simulink model "lunwen_huitu"  (R2020b)
settings: Solver=ode45  StartTime=0.0  StopTime=2  RelTol=1e-3  EnableMultiTasking=on
values from neighbouring files (symbols this model uses):
  alphar = poly2sym(y3,t)    [lpv_model.m]
  hr = poly2sym(y6,t)    [lpv_model.m]
  miur = poly2sym(y2,t)    [lpv_model.m]
  qr = poly2sym(y4,t)    [lpv_model.m]
  Vr = poly2sym(y1,t)    [lpv_model.m]
  xr = poly2sym(y5,t)    [lpv_model.m]    (also in xr(0.0.01.2).mat = [9.97354758391 9.97900733809 9.98348279699 9.98718538751 9.9)
settings Model: Creator=YuXiaozhi  LastModifiedBy=Eric
settings DataIOCC: LimitDataPoints=on  SaveFormat=Array  ReturnWorkspaceOutputs=off
settings OptimizationCC: LifeSpan=inf
settings DebuggingCC: SolverPrmCheckMsg=warning  SFUnexpectedBacktrackingDiag=warning  SFNoUnconditionalDefaultTransitionDiag=warning  ArithmeticOperatorsInVariantConditions=warning
settings HardwareCC: ProdBitPerPointer=32  ProdBitPerSizeT=32  ProdBitPerPtrDiffT=32  ProdLargestAtomicFloat=None  ProdIntDivRoundTo=Undefined  ProdEndianess=Unspecified  ProdWordSize=32  ProdHWDeviceType=32-bit Generic
settings ModelReferenceCC: PropagateSignalLabelsOutOfModel=off
settings SFSimCC: SimUseLocalCustomCode=off  CustomCodeUndefinedFunction=UseInterfaceOnly
settings RTWCC: RTWUseLocalCustomCode=off
settings CodeAppCC: StateflowObjectComments=on
settings GRTTargetCC: TargetLangStandard=C89/C90 (ANSI)
settings ConfigComp: CovMetricSettings=dw  CovSaveCumulativeToWorkspaceVar=on  CovSaveSingleToWorkspaceVar=on  CovExternalEMLEnable=off  CovSFcnEnable=off

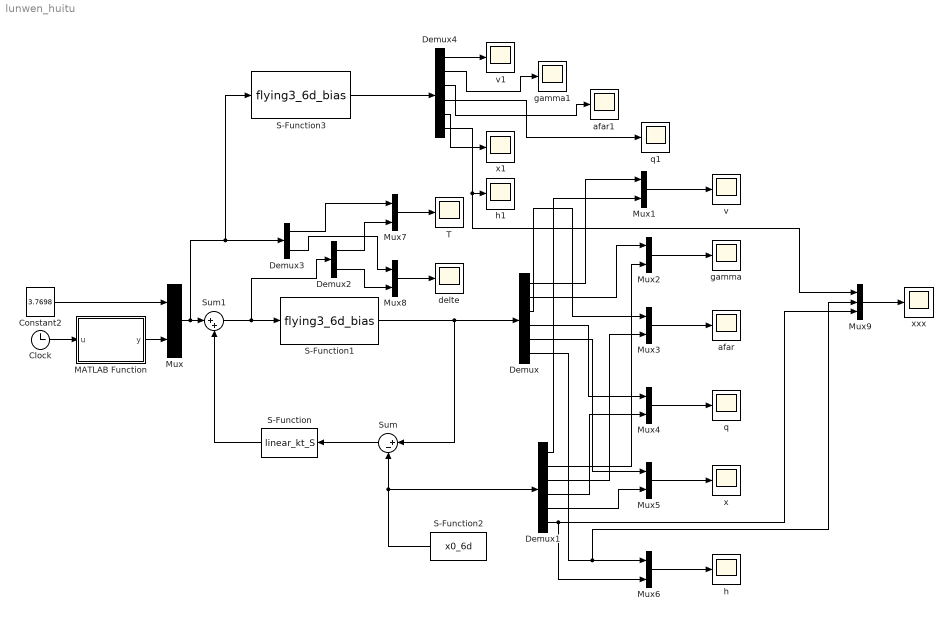
== system lunwen_huitu ==
  Clock : Clock
  Constant2 : Constant  Value=3.7698
  Demux : Demux  Outputs=6
  Demux1 : Demux  Outputs=6
  Demux2 : Demux  Outputs=2
  Demux3 : Demux  Outputs=2
  Demux4 : Demux  Outputs=6
  MATLAB Function : MATLAB Function  TreatAsAtomicUnit=on
  Mux{,1..8} (9 alike) : Mux  Inputs=2
  Mux9 : Mux  Inputs=3
  S-Function : S-Function  FunctionName=linear_kt_S  Parameters=Kall  SFunctionDeploymentMode=off  EnableBusSupport=off
  S-Function1 : S-Function  FunctionName=flying3_6d_bias  SFunctionDeploymentMode=off  EnableBusSupport=off
  S-Function2 : S-Function  FunctionName=x0_6d  Parameters=Vr,miur,alphar,qr,xr,hr  SFunctionDeploymentMode=off  EnableBusSupport=off
  S-Function3 : S-Function  FunctionName=flying3_6d_bias  SFunctionDeploymentMode=off  EnableBusSupport=off
  Sum : Sum  Inputs=|+-
  Sum1 : Sum  Inputs=|++
  T : Scope
  afar : Scope
  afar1 : Scope
  delte : Scope
  gamma : Scope
  gamma1 : Scope
  h : Scope
  h1 : Scope
  q : Scope
  q1 : Scope
  v : Scope
  v1 : Scope
  x : Scope
  x1 : Scope
  xxx : Scope
  wires:
  S-Function1/1 -> Sum/1, Demux/1
  S-Function2/1 -> Demux1/1, Sum/2
  Sum/1 -> S-Function/1
  Clock/1 -> MATLAB Function/1(u)
  Constant2/1 -> Mux/1
  MATLAB Function/1(y) -> Mux/2
  Mux/1 -> S-Function3/1, Demux3/1, Sum1/1
  Sum1/1 -> Demux2/1, S-Function1/1
  Demux2/1 -> Mux7/2
  Demux2/2 -> Mux8/2
  Mux7/1 -> T/1
  Mux8/1 -> delte/1
  Demux3/1 -> Mux7/1
  Demux3/2 -> Mux8/1
  Demux/1 -> Mux1/1
  Demux/2 -> Mux2/1
  Demux/3 -> Mux3/1
  Demux/4 -> Mux4/1
  Demux/5 -> Mux5/1
  Demux/6 -> Mux9/2, Mux6/1
  Demux1/1 -> Mux1/2
  Demux1/2 -> Mux2/2
  Demux1/3 -> Mux3/2
  Demux1/4 -> Mux4/2
  Demux1/5 -> Mux5/2
  Demux1/6 -> Mux9/3, Mux6/2
  Mux1/1 -> v/1
  Mux2/1 -> gamma/1
  Mux3/1 -> afar/1
  Mux4/1 -> q/1
  Mux5/1 -> x/1
  Mux6/1 -> h/1
  S-Function3/1 -> Demux4/1
  Demux4/1 -> v1/1
  Demux4/2 -> gamma1/1
  Demux4/3 -> afar1/1
  Demux4/4 -> q1/1
  Demux4/5 -> x1/1
  Demux4/6 -> Mux9/1, h1/1
  Mux9/1 -> xxx/1
  S-Function/1 -> Sum1/2

== matlab function lunwen_huitu/MATLAB Function ==
  data: u input; y output
function y = fcn(u)
if u<0.3
    y=-(11+(u)/0.3*22)/180*pi;
else if u>=0.3&&u<0.5
        y=-(33+(u-0.3)/0.2*15)/180*pi;
else if u>=0.5&&u<0.7
        y=-(33+15-(u-0.5)/0.2*30)/180*pi;   
    else
        y=-(18)/180*pi;
    end
    end
end
